simulink model "myproject_task"  (Simulink 3.00)
libraries: genlib x2, mathlib x1

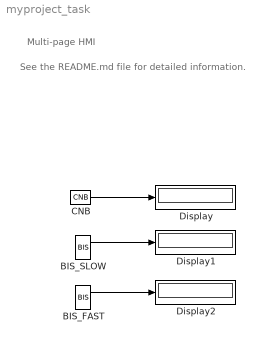
== system myproject_task ==
  note: See the README.md file for detailed information.
  note: Multi-page HMI
  BIS_FAST : genlib/BIS  Y0=off  t1=0.5  t2=1.0  t3=0  t4=4  t5=5  t6=6  t7=7  t8=8  RPT=on
  BIS_SLOW : genlib/BIS  Y0=off  t1=2  t2=4  t3=0  t4=4  t5=5  t6=6  t7=7  t8=8  RPT=on
  CNB : mathlib/CNB  YCN=on
  Display : Display
      settings: Format=Best fit
  Display1 : Display
      settings: Format=Best fit
  Display2 : Display
      settings: Format=Best fit
  wires:
  BIS_FAST/1 -> Display2/1
  BIS_SLOW/1 -> Display1/1
  CNB/1 -> Display/1
